simulink model "fifth_equation_test"  (R2017b)
settings: Solver=VariableStepAuto  StartTime=0.0  StopTime=5  RelTol=1e-3
undefined symbols (not defined in the file): quad
libraries: NLGCToolbox x2
settings Model: Creator=hoang  LastModifiedBy=hoang

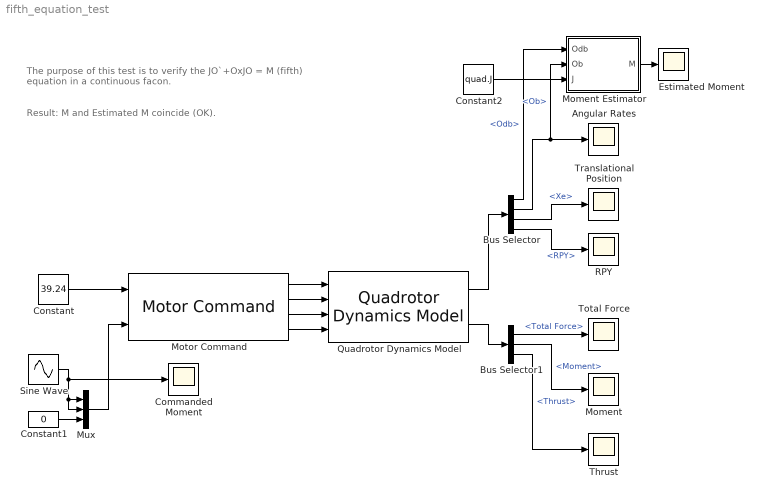
== system fifth_equation_test ==
  note: The purpose of this test is to verify the JO`+OxJO = M (fifth) equation in a continuous facon.
  note: Result: M and Estimated M coincide (OK).
  Angular Rates : Scope
  Bus Selector : BusSelector  OutputSignals=Odb,Ob,Xe,RPY
  Bus Selector1 : BusSelector  OutputSignals=Total Force,Moment,Thrust
  Commanded Moment : Scope
  Constant : Constant  Value=39.24
  Constant1 : Constant  Value=0
  Constant2 : Constant  Value=quad.J
  Estimated Moment : Scope
  Moment : Scope
  Moment Estimator : MATLAB Function  TreatAsAtomicUnit=on
  Motor Command : NLGCToolbox/Motor Command  quadrotor=quad
      settings: SourceProductName=Thinh - NLGC for Quadrotor
  Mux : Mux  Inputs=3
  Quadrotor Dynamics Model : NLGCToolbox/Quadrotor Dynamics Model  xinit=[0 0 -4]  quadrotor=quad
      settings: SourceProductName=Thinh - NLGC for Quadrotor
  RPY : Scope
  Sine Wave : Sin  Amplitude=0.005  Frequency=2*pi/5  SampleTime=0
  Thrust : Scope
  Total Force : Scope
  Translational Position : Scope
  wires:
  Motor Command/1 -> Quadrotor Dynamics Model/1
  Motor Command/2 -> Quadrotor Dynamics Model/2
  Motor Command/3 -> Quadrotor Dynamics Model/3
  Motor Command/4 -> Quadrotor Dynamics Model/4
  Constant/1 -> Motor Command/1
  Quadrotor Dynamics Model/1 -> Bus Selector/1
  Bus Selector/3 -> Translational Position/1  "<Xe>"
  Bus Selector/4 -> RPY/1  "<RPY>"
  Quadrotor Dynamics Model/2 -> Bus Selector1/1
  Bus Selector1/1 -> Total Force/1  "<Total Force>"
  Bus Selector1/2 -> Moment/1  "<Moment>"
  Mux/1 -> Motor Command/2
  Sine Wave/1 -> Commanded Moment/1, Mux/2, Mux/1
  Bus Selector1/3 -> Thrust/1  "<Thrust>"
  Constant1/1 -> Mux/3
  Bus Selector/2 -> Moment Estimator/2(Ob), Angular Rates/1  "<Ob>"
  Bus Selector/1 -> Moment Estimator/1(Odb)  "<Odb>"
  Moment Estimator/1(M) -> Estimated Moment/1
  Constant2/1 -> Moment Estimator/3(J)

== matlab function fifth_equation_test/Moment Estimator ==
  data: M output size=[3 1]; Odb input size=[3 1]; Ob input size=[3 1]; J input size=[3 3]
function M = fcn(Odb,Ob,J)
M = J*Odb + hat(Ob)*(J*Ob);
